simulink model "scheme"  (R2021a)
settings: Solver=VariableStepAuto  StartTime=0.0  StopTime=150  MaxStep=0.5  RelTol=1e-3
libraries: simulink x1
settings Model: Creator=mirlan  LastModifiedBy=mirlan

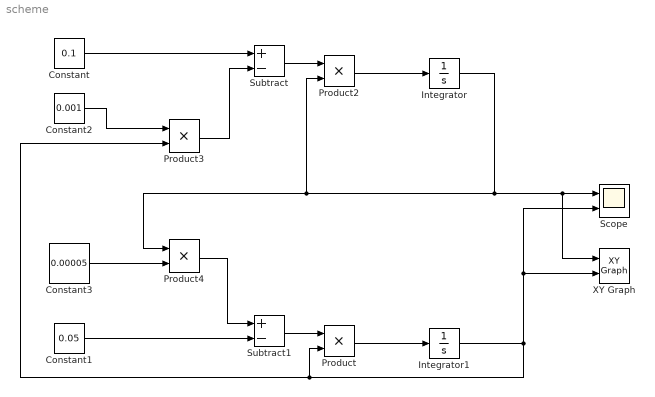
== system scheme ==
  Constant : Constant  Value=0.1
  Constant1 : Constant  Value=0.05
  Constant2 : Constant  Value=0.001
  Constant3 : Constant  Value=0.00005
  Integrator : Integrator  InitialCondition=50
  Integrator1 : Integrator  InitialCondition=120
  Product{,2..4} (4 alike) : Product
  Scope : Scope  NumInputPorts=2
  Subtract : Sum  Inputs=+-
  Subtract1 : Sum  Inputs=+-
  XY Graph : simulink/Sinks/XY Graph  xmin=-100  xmax=5000  ymin=-100  ymax=500  st=-1
  wires:
  Integrator/1 -> Scope/1, XY Graph/1, Product2/2, Product4/1
  Integrator1/1 -> XY Graph/2, Scope/2, Product/2, Product3/2
  Product4/1 -> Subtract1/1
  Constant3/1 -> Product4/2
  Constant/1 -> Subtract/1
  Constant2/1 -> Product3/1
  Product3/1 -> Subtract/2
  Constant1/1 -> Subtract1/2
  Subtract1/1 -> Product/1
  Product/1 -> Integrator1/1
  Product2/1 -> Integrator/1
  Subtract/1 -> Product2/1
